simulink library "lka"  (Simulink 8.2)
settings: Solver=ode1  StartTime=0.0  StopTime=Inf  FixedStep=0.001  RelTol=1e-3
PostLoadFcn:
  | , if any(exist('dsrtsu_mdlpostloadfcn', 'file') == [2, 3, 6]), try dsrtsu_mdlpostloadfcn('Execute', bdroot); catch fprintf('Error in PostLoadFcn (dsrtsu_mdlpostloadfcn) for model "%s":\n %s\n', bdroot, lasterr); end, end,
undefined symbols (not defined in the file or in its folder): ALFC_VehSpd_X_kph, ALKA_LatSpd_X_mps, ALKA_VehSpd_X_kph, ENUM_LKASTATE_ADASFAILURE, ENUM_LKASTATE_DISABLED, ENUM_LKASTATE_EPSRECOVERYPENDING, ENUM_LKASTATE_LEFTASSISTING, ENUM_LKASTATE_OFF, ENUM_LKASTATE_OPERATIONAL, ENUM_LKASTATE_RIGHTASSISTING, ENUM_LKASTATE_STANDBY, FALSE, KAPP_StrCenterOffset_deg, KAPP_VehicleWidth_m, KAPP_Wheel2SteerRatio_rat, KAPP_WheelBase_m, KLKA_BaseTqReqMax_Nm, KLKA_BaseTqReqMin_Nm, KLKA_IGainLowerLimit_rad, KLKA_IGainUpperLimit_rad, KLKA_LKATqReqMax_Nm, KLKA_LKATqReqMin_Nm, KLKA_TargetPointShift_m, MLFC_KusCoeff_rat, MLKA_ControlGain_rat, MLKA_KgainRatio_rat, MLKA_LookAheadDist_Y_m, TRUE
libraries: hcu_lib x8, simulink x2
settings Model: DSRTSU_INTERNAL_RTI_VER=450  DSRTSU_INTERNAL_RTI_TYPE=rti1401  RTICANMMDATA=struct('GeneralSetupData',struct('modelroot','C:\ADAS\trunk\ADAS_Softwares\HTDragon\software\sw_development\arch\app\lka','generalsettings',struct('filesettings',struct('destfolder',struct('Name','RTICANMM_FILES','Check',1),'buildfolder',struct('Name','.','Check',1),'AbsDestfolder',struct('Name','C:\ADAS\trunk\ADAS_Softwares\HTDragon\software\sw_development\arch\app\lka\RTICANMM_FILES'),'AbsBuildfolder',struct('Name','C:\ADAS\trunk\ADAS_Softwares\HTDragon\software\sw_development\arch\app\lka'))),'options',struct('addpaths',1,'rmpaths',1,'addtrcexclusion',logical(1),'cannavigator',struct('checkmonitoring',0),'show_usrtrc',0,'use_usrtrc',0),'advanced',struct('options',[1 1 1 1 1 1 1 1 1 1 1 1 1 1 1 1 1 1 1 1 1 1 1 1 1 1 1 1 1 1 1 1 1 1 1 1 1 1 1 1 1 1 1 1 1 1 1 1 1 1 1 1 1 1 1 1 1 1 1 1 1 1 1 1 1 1 1 1 1 1 1 1 1 1 1 1 1 1 1 1 1 1 1 1 1 1 1 1 1 1 1 1 1 1 1 1 1 1 1 1]),'MPSetup',{{}},'modelname','lka','block','lka'))  DSRTSU_INTERNAL_RTIFPGA=40  Creator=14014  LastModifiedBy=13192

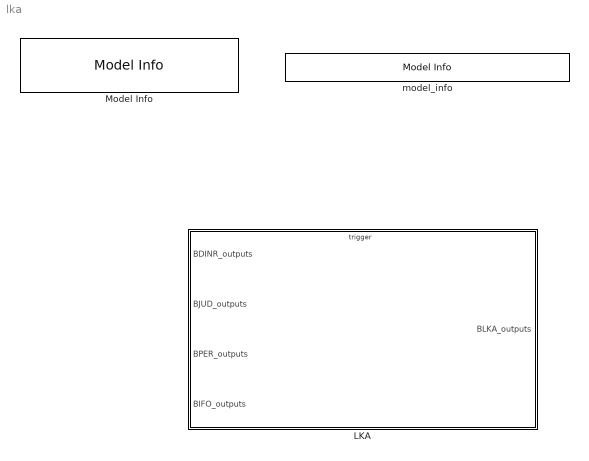
== system lka ==
  LKA : Subsystem
  Model Info : simulink/Model-Wide Utilities/Model Info  InitialBlockCM=None  BlockCM=None  Frame=on  DisplayStringWithTags=|  HorizontalTextAlignment=Left  LeftAlignmentValue=0.02  SourceBlockDiagram=lka  TagMaxNumber=20
      | Model Version        : %<ModelVersion>
      | Creator                   : %<Creator>
      | Last Modified by    : %<LastModifiedBy>
  model_info : simulink/Model-Wide Utilities/Model Info  InitialBlockCM=None  BlockCM=None  Frame=on  DisplayStringWithTags=$Id: lka.mdl 1622 2017-09-21 01:44:11Z bcluan $  HorizontalTextAlignment=Center  LeftAlignmentValue=0.5  SourceBlockDiagram=lka  TagMaxNumber=20

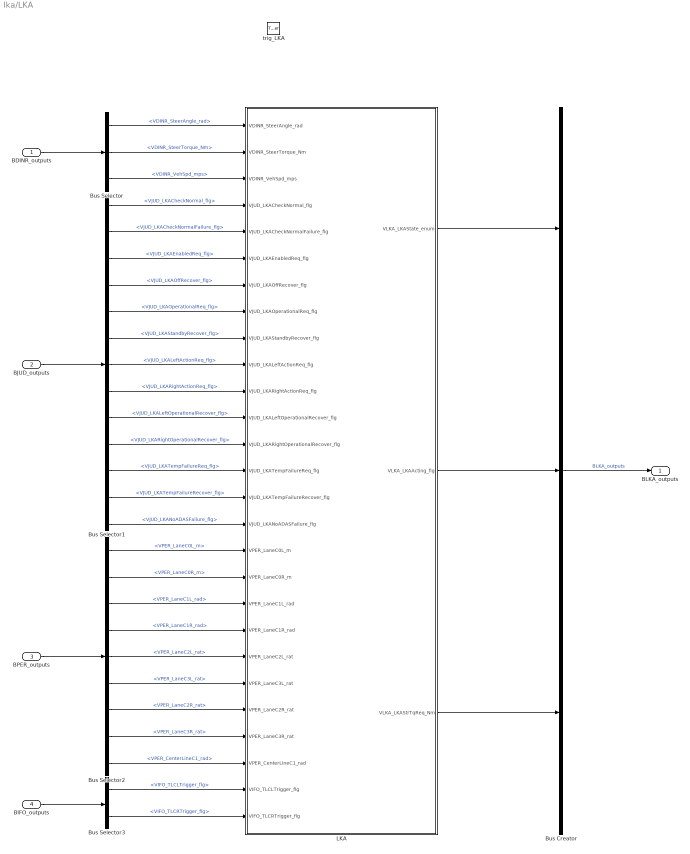
== system lka/LKA ==
  BDINR_outputs : Inport  OutDataTypeStr=Bus: BDINR_outputs
  BJUD_outputs : Inport  Port=2  OutDataTypeStr=Bus: BJUD_outputs
  BPER_outputs : Inport  Port=3  OutDataTypeStr=Bus: BPER_outputs
  BIFO_outputs : Inport  Port=4  OutDataTypeStr=Bus: BIFO_outputs
  trig_LKA : TriggerPort  TriggerType=function-call
      settings: AttributesFormatString=State = %<StatesWhenEnabling>
  Bus Creator : BusCreator  Inputs=3  OutDataTypeStr=Bus: BLKA_outputs
  Bus Selector : BusSelector  OutputSignals=VDINR_SteerAngle_rad,VDINR_SteerTorque_Nm,VDINR_VehSpd_mps
  Bus Selector1 : BusSelector  OutputSignals=VJUD_LKACheckNormal_flg,VJUD_LKACheckNormalFailure_flg,VJUD_LKAEnabledReq_flg,VJUD_LKAOffRecover_flg,VJUD_LKAOperationalReq_flg,VJUD_LKAStandbyRecover_flg,VJUD_LKALeftActionReq_flg,VJUD_LKARightActionReq_flg,VJUD_LKALeftOperationalRecover_flg,VJUD_LKARightOperationalRecover_flg,VJUD_LKATempFailureReq_flg,VJUD_LKATempFailureRecover_flg,VJUD_LKANoADASFailure_flg
  Bus Selector2 : BusSelector  OutputSignals=VPER_LaneC0L_m,VPER_LaneC0R_m,VPER_LaneC1L_rad,VPER_LaneC1R_rad,VPER_LaneC2L_rat,VPER_LaneC3L_rat,VPER_LaneC2R_rat,VPER_LaneC3R_rat,VPER_CenterLineC1_rad
  Bus Selector3 : BusSelector  OutputSignals=VIFO_TLCLTrigger_flg,VIFO_TLCRTrigger_flg
  LKA : Subsystem
  BLKA_outputs : Outport  OutDataTypeStr=Bus: BLKA_outputs
  wires:
  Bus Creator/1 -> BLKA_outputs/1  "BLKA_outputs"
  BDINR_outputs/1 -> Bus Selector/1
  BPER_outputs/1 -> Bus Selector2/1
  BJUD_outputs/1 -> Bus Selector1/1
  BIFO_outputs/1 -> Bus Selector3/1
  LKA/2(VLKA_LKAActing_flg) -> Bus Creator/2
  LKA/3(VLKA_LKAStrTqReq_Nm) -> Bus Creator/3
  LKA/1(VLKA_LKAState_enum) -> Bus Creator/1
  Bus Selector1/1 -> LKA/4(VJUD_LKACheckNormal_flg)  "<VJUD_LKACheckNormal_flg>"
  Bus Selector1/3 -> LKA/6(VJUD_LKAEnabledReq_flg)  "<VJUD_LKAEnabledReq_flg>"
  Bus Selector1/4 -> LKA/7(VJUD_LKAOffRecover_flg)  "<VJUD_LKAOffRecover_flg>"
  Bus Selector1/5 -> LKA/8(VJUD_LKAOperationalReq_flg)  "<VJUD_LKAOperationalReq_flg>"
  Bus Selector1/6 -> LKA/9(VJUD_LKAStandbyRecover_flg)  "<VJUD_LKAStandbyRecover_flg>"
  Bus Selector1/7 -> LKA/10(VJUD_LKALeftActionReq_flg)  "<VJUD_LKALeftActionReq_flg>"
  Bus Selector1/8 -> LKA/11(VJUD_LKARightActionReq_flg)  "<VJUD_LKARightActionReq_flg>"
  Bus Selector1/9 -> LKA/12(VJUD_LKALeftOperationalRecover_flg)  "<VJUD_LKALeftOperationalRecover_flg>"
  Bus Selector1/10 -> LKA/13(VJUD_LKARightOperationalRecover_flg)  "<VJUD_LKARightOperationalRecover_flg>"
  Bus Selector1/11 -> LKA/14(VJUD_LKATempFailureReq_flg)  "<VJUD_LKATempFailureReq_flg>"
  Bus Selector1/12 -> LKA/15(VJUD_LKATempFailureRecover_flg)  "<VJUD_LKATempFailureRecover_flg>"
  Bus Selector1/13 -> LKA/16(VJUD_LKANoADASFailure_flg)  "<VJUD_LKANoADASFailure_flg>"
  Bus Selector2/8 -> LKA/24(VPER_LaneC3R_rat)  "<VPER_LaneC3R_rat>"
  Bus Selector2/7 -> LKA/23(VPER_LaneC2R_rat)  "<VPER_LaneC2R_rat>"
  Bus Selector2/3 -> LKA/19(VPER_LaneC1L_rad)  "<VPER_LaneC1L_rad>"
  Bus Selector2/2 -> LKA/18(VPER_LaneC0R_m)  "<VPER_LaneC0R_m>"
  Bus Selector2/1 -> LKA/17(VPER_LaneC0L_m)  "<VPER_LaneC0L_m>"
  Bus Selector2/4 -> LKA/20(VPER_LaneC1R_rad)  "<VPER_LaneC1R_rad>"
  Bus Selector2/6 -> LKA/22(VPER_LaneC3L_rat)  "<VPER_LaneC3L_rat>"
  Bus Selector2/5 -> LKA/21(VPER_LaneC2L_rat)  "<VPER_LaneC2L_rat>"
  Bus Selector2/9 -> LKA/25(VPER_CenterLineC1_rad)  "<VPER_CenterLineC1_rad>"
  Bus Selector3/1 -> LKA/26(VIFO_TLCLTrigger_flg)  "<VIFO_TLCLTrigger_flg>"
  Bus Selector3/2 -> LKA/27(VIFO_TLCRTrigger_flg)  "<VIFO_TLCRTrigger_flg>"
  Bus Selector/1 -> LKA/1(VDINR_SteerAngle_rad)  "<VDINR_SteerAngle_rad>"
  Bus Selector/2 -> LKA/2(VDINR_SteerTorque_Nm)  "<VDINR_SteerTorque_Nm>"
  Bus Selector/3 -> LKA/3(VDINR_VehSpd_mps)  "<VDINR_VehSpd_mps>"
  Bus Selector1/2 -> LKA/5(VJUD_LKACheckNormalFailure_flg)  "<VJUD_LKACheckNormalFailure_flg>"

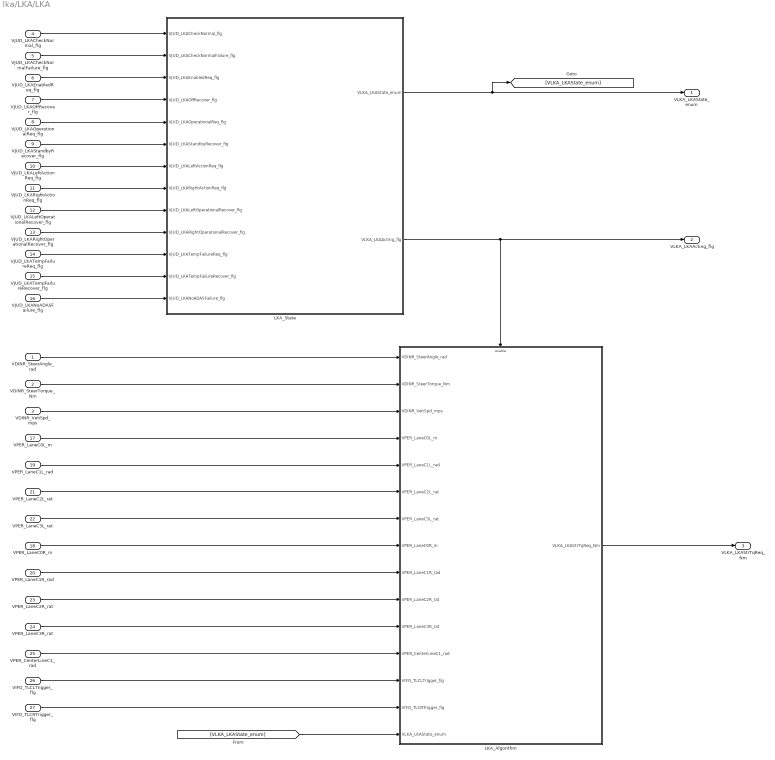
== system lka/LKA/LKA ==
  VDINR_SteerAngle_rad : Inport
  VDINR_SteerTorque_Nm : Inport  Port=2
  VDINR_VehSpd_mps : Inport  Port=3
  VJUD_LKACheckNormal_flg : Inport  Port=4
  VJUD_LKACheckNormalFailure_flg : Inport  Port=5
  VJUD_LKAEnabledReq_flg : Inport  Port=6
  VJUD_LKAOffRecover_flg : Inport  Port=7
  VJUD_LKAOperationalReq_flg : Inport  Port=8
  VJUD_LKAStandbyRecover_flg : Inport  Port=9
  VJUD_LKALeftActionReq_flg : Inport  Port=10
  VJUD_LKARightActionReq_flg : Inport  Port=11
  VJUD_LKALeftOperationalRecover_flg : Inport  Port=12
  VJUD_LKARightOperationalRecover_flg : Inport  Port=13
  VJUD_LKATempFailureReq_flg : Inport  Port=14
  VJUD_LKATempFailureRecover_flg : Inport  Port=15
  VJUD_LKANoADASFailure_flg : Inport  Port=16
  VPER_LaneC0L_m : Inport  Port=17
  VPER_LaneC0R_m : Inport  Port=18
  VPER_LaneC1L_rad : Inport  Port=19
  VPER_LaneC1R_rad : Inport  Port=20
  VPER_LaneC2L_rat : Inport  Port=21
  VPER_LaneC3L_rat : Inport  Port=22
  VPER_LaneC2R_rat : Inport  Port=23
  VPER_LaneC3R_rat : Inport  Port=24
  VPER_CenterLineC1_rad : Inport  Port=25
  VIFO_TLCLTrigger_flg : Inport  Port=26
  VIFO_TLCRTrigger_flg : Inport  Port=27
  LKA_Algorithm : Subsystem
  LKA_State : Stateflow chart  TreatAsAtomicUnit=on
  VLKA_LKAState_enum : Outport  OutputWhenDisabled=reset  InitialOutput=[0]
  VLKA_LKAActing_flg : Outport  Port=2  OutputWhenDisabled=reset  InitialOutput=[0]
  VLKA_LKAStrTqReq_Nm : Outport  Port=3  OutputWhenDisabled=reset  InitialOutput=[0]
  wires:
  VJUD_LKACheckNormal_flg/1 -> LKA_State/1(VJUD_LKACheckNormal_flg)
  VJUD_LKAEnabledReq_flg/1 -> LKA_State/3(VJUD_LKAEnabledReq_flg)
  VJUD_LKAOffRecover_flg/1 -> LKA_State/4(VJUD_LKAOffRecover_flg)
  VJUD_LKAOperationalReq_flg/1 -> LKA_State/5(VJUD_LKAOperationalReq_flg)
  VJUD_LKAStandbyRecover_flg/1 -> LKA_State/6(VJUD_LKAStandbyRecover_flg)
  VJUD_LKALeftActionReq_flg/1 -> LKA_State/7(VJUD_LKALeftActionReq_flg)
  VJUD_LKALeftOperationalRecover_flg/1 -> LKA_State/9(VJUD_LKALeftOperationalRecover_flg)
  VJUD_LKATempFailureReq_flg/1 -> LKA_State/11(VJUD_LKATempFailureReq_flg)
  VJUD_LKATempFailureRecover_flg/1 -> LKA_State/12(VJUD_LKATempFailureRecover_flg)
  VJUD_LKANoADASFailure_flg/1 -> LKA_State/13(VJUD_LKANoADASFailure_flg)
  LKA_State/1(VLKA_LKAState_enum) -> [VLKA_LKAState_enum], VLKA_LKAState_enum/1
  LKA_State/2(VLKA_LKAActing_flg) -> VLKA_LKAActing_flg/1, LKA_Algorithm/Enable
  LKA_Algorithm/1(VLKA_LKAStrTqReq_Nm) -> VLKA_LKAStrTqReq_Nm/1
  VDINR_VehSpd_mps/1 -> LKA_Algorithm/3(VDINR_VehSpd_mps)
  VIFO_TLCLTrigger_flg/1 -> LKA_Algorithm/13(VIFO_TLCLTrigger_fig)
  VIFO_TLCRTrigger_flg/1 -> LKA_Algorithm/14(VIFO_TLCRTrigger_fig)
  VDINR_SteerAngle_rad/1 -> LKA_Algorithm/1(VDINR_SteerAngle_rad)
  VDINR_SteerTorque_Nm/1 -> LKA_Algorithm/2(VDINR_SteerTorque_Nm)
  VJUD_LKARightActionReq_flg/1 -> LKA_State/8(VJUD_LKARightActionReq_flg)
  VJUD_LKARightOperationalRecover_flg/1 -> LKA_State/10(VJUD_LKARightOperationalRecover_flg)
  VPER_LaneC0L_m/1 -> LKA_Algorithm/4(VPER_LaneC0L_m)
  VPER_LaneC1L_rad/1 -> LKA_Algorithm/5(VPER_LaneC1L_rad)
  VPER_LaneC0R_m/1 -> LKA_Algorithm/8(VPER_LaneC0R_m)
  VPER_LaneC1R_rad/1 -> LKA_Algorithm/9(VPER_LaneC1R_rad)
  VPER_LaneC2L_rat/1 -> LKA_Algorithm/6(VPER_LaneC2L_rat)
  VPER_LaneC3L_rat/1 -> LKA_Algorithm/7(VPER_LaneC3L_rat)
  VPER_LaneC2R_rat/1 -> LKA_Algorithm/10(VPER_LaneC2R_rat)
  VPER_LaneC3R_rat/1 -> LKA_Algorithm/11(VPER_LaneC3R_rat)
  VPER_CenterLineC1_rad/1 -> LKA_Algorithm/12(VPER_CenterLineC1_rad)
  [VLKA_LKAState_enum] -> LKA_Algorithm/15(VLKA_LKAState_enum)
  VJUD_LKACheckNormalFailure_flg/1 -> LKA_State/2(VJUD_LKACheckNormalFailure_flg)

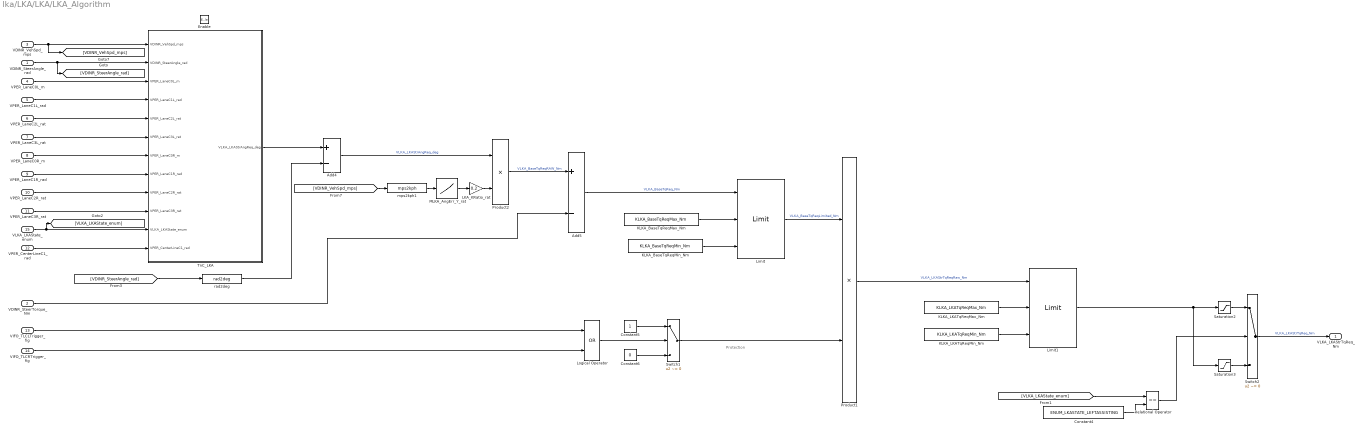
== system lka/LKA/LKA/LKA_Algorithm ==
  note: Protection
  VDINR_SteerAngle_rad : Inport
  VDINR_SteerTorque_Nm : Inport  Port=2
  VDINR_VehSpd_mps : Inport  Port=3
  VPER_LaneC0L_m : Inport  Port=4
  VPER_LaneC1L_rad : Inport  Port=5
  VPER_LaneC2L_rat : Inport  Port=6
  VPER_LaneC3L_rat : Inport  Port=7
  VPER_LaneC0R_m : Inport  Port=8
  VPER_LaneC1R_rad : Inport  Port=9
  VPER_LaneC2R_rat : Inport  Port=10
  VPER_LaneC3R_rat : Inport  Port=11
  VPER_CenterLineC1_rad : Inport  Port=12
  VIFO_TLCLTrigger_fig : Inport  Port=13
  VIFO_TLCRTrigger_fig : Inport  Port=14
  VLKA_LKAState_enum : Inport  Port=15
  Enable : EnablePort  StatesWhenEnabling=reset
  Add4 : Sum  Inputs=+-
  Add5 : Sum  Inputs=+-
  Constant4 : Constant  Value=ENUM_LKASTATE_LEFTASSISTING
  Constant5 : Constant  OutDataTypeStr=single
  Constant6 : Constant  Value=0  OutDataTypeStr=single
  KLKA_BaseTqReqMax_Nm : Constant  Value=KLKA_BaseTqReqMax_Nm  OutDataTypeStr=single
  KLKA_BaseTqReqMin_Nm : Constant  Value=KLKA_BaseTqReqMin_Nm  OutDataTypeStr=single
  KLKA_LKATqReqMax_Nm : Constant  Value=KLKA_LKATqReqMax_Nm  OutDataTypeStr=single
  KLKA_LKATqReqMin_Nm : Constant  Value=KLKA_LKATqReqMin_Nm  OutDataTypeStr=single
  LKA_KRatio_rat : Gain  Gain=0.2
  Limit : hcu_lib/Limit  SystemSampleTime=-1
  Limit1 : hcu_lib/Limit  SystemSampleTime=-1
  Logical Operator : Logic  Operator=OR  AllPortsSameDT=off  OutDataTypeStr=boolean
  MLKA_AngErr_Y_rat : Lookup  InputValues=[10:10:120]  Table=[1 1 1 1 1 1 1 1 1 1 1 1]  LookUpMeth=Interpolation-Use End Values
      settings: AttributesFormatString=%<InputValues>\n%<Table>
  Product1 : Product  RndMeth=Zero
  Product2 : Product
  Relational Operator : RelationalOperator  Operator===  OutDataTypeStr=boolean
  Saturation2 : Saturate  UpperLimit=0  LowerLimit=-inf
      settings: AttributesFormatString=|
      | %<UpperLimit>
      | %<LowerLimit>
  Saturation3 : Saturate  UpperLimit=inf  LowerLimit=0
      settings: AttributesFormatString=|
      | %<UpperLimit>
      | %<LowerLimit>
  Switch1 : Switch  Criteria=u2 ~= 0
  Switch2 : Switch  Criteria=u2 ~= 0
  TnC_LKA : Subsystem  TreatAsAtomicUnit=on
  mps2kph1 : hcu_lib/mps2kph
  rad2deg : hcu_lib/rad2deg
  VLKA_LKAStrTqReq_Nm : Outport  OutputWhenDisabled=reset  InitialOutput=[0]
  wires:
  Constant6/1 -> Switch1/3
  VIFO_TLCLTrigger_fig/1 -> Logical Operator/1
  VIFO_TLCRTrigger_fig/1 -> Logical Operator/2
  Logical Operator/1 -> Switch1/2
  Constant5/1 -> Switch1/1
  VDINR_SteerTorque_Nm/1 -> Add5/2
  VDINR_VehSpd_mps/1 -> [VDINR_VehSpd_mps], TnC_LKA/1(VDINR_VehSpd_mps)
  [VDINR_SteerAngle_rad] -> rad2deg/1
  TnC_LKA/1(VLKA_LKAStrAngReq_deg) -> Add4/1
  rad2deg/1 -> Add4/2
  Add4/1 -> Product2/1  "VLKA_LKAStrAngReq_deg"
  Product2/1 -> Add5/1  "VLKA_BaseTqReqRAW_Nm"
  Limit/1 -> Product1/1  "VLKA_BaseTqReqLimited_Nm"
  KLKA_BaseTqReqMax_Nm/1 -> Limit/2
  KLKA_BaseTqReqMin_Nm/1 -> Limit/3
  Add5/1 -> Limit/1  "VLKA_BaseTqReq_Nm"
  VDINR_SteerAngle_rad/1 -> [VDINR_SteerAngle_rad], TnC_LKA/2(VDINR_SteerAngle_rad)
  VPER_LaneC0L_m/1 -> TnC_LKA/3(VPER_LaneC0L_m)
  VPER_LaneC1L_rad/1 -> TnC_LKA/4(VPER_LaneC1L_rad)
  VPER_LaneC2L_rat/1 -> TnC_LKA/5(VPER_LaneC2L_rat)
  VPER_LaneC3L_rat/1 -> TnC_LKA/6(VPER_LaneC3L_rat)
  VPER_LaneC0R_m/1 -> TnC_LKA/7(VPER_LaneC0R_m)
  VPER_LaneC1R_rad/1 -> TnC_LKA/8(VPER_LaneC1R_rad)
  VPER_LaneC2R_rat/1 -> TnC_LKA/9(VPER_LaneC2R_rat)
  VPER_LaneC3R_rat/1 -> TnC_LKA/10(VPER_LaneC3R_rat)
  VLKA_LKAState_enum/1 -> [VLKA_LKAState_enum], TnC_LKA/11(VLKA_LKAState_enum)
  KLKA_LKATqReqMax_Nm/1 -> Limit1/2
  KLKA_LKATqReqMin_Nm/1 -> Limit1/3
  Product1/1 -> Limit1/1  "VLKA_LKAStrTqReqRaw_Nm"
  MLKA_AngErr_Y_rat/1 -> LKA_KRatio_rat/1
  mps2kph1/1 -> MLKA_AngErr_Y_rat/1
  [VDINR_VehSpd_mps] -> mps2kph1/1
  VPER_CenterLineC1_rad/1 -> TnC_LKA/12(VPER_CenterLineC1_rad)
  Switch1/1 -> Product1/2
  LKA_KRatio_rat/1 -> Product2/2
  Limit1/1 -> Saturation3/1, Saturation2/1
  Saturation2/1 -> Switch2/1
  Saturation3/1 -> Switch2/3
  Switch2/1 -> VLKA_LKAStrTqReq_Nm/1  "VLKA_LKAStrTqReq_Nm"
  [VLKA_LKAState_enum] -> Relational Operator/1
  Constant4/1 -> Relational Operator/2
  Relational Operator/1 -> Switch2/2

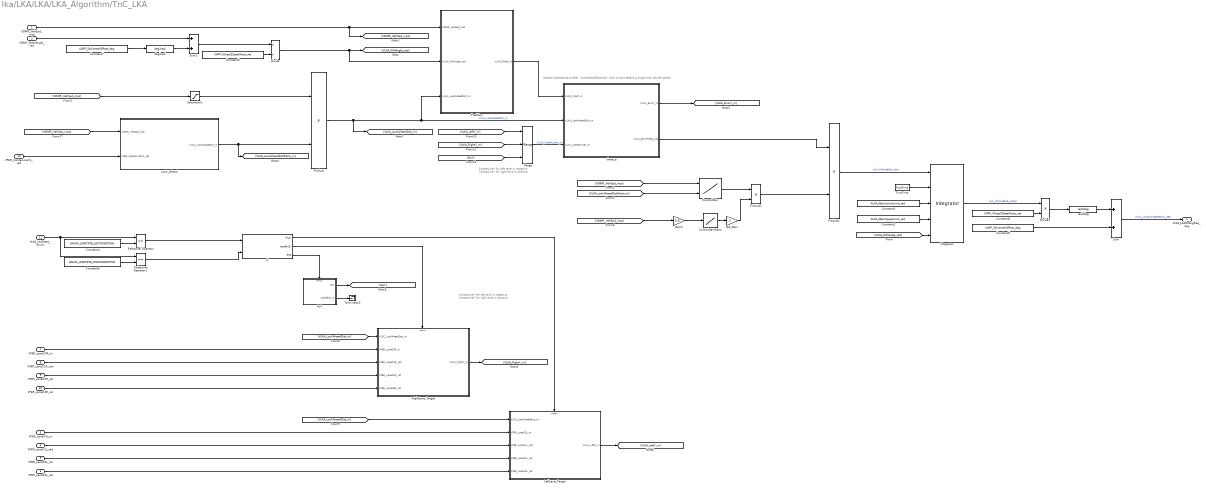
== system lka/LKA/LKA/LKA_Algorithm/TnC_LKA ==
  note: CenterLineY for left lane is negative
      | CenterLineY for right lane is positive
  note: Lateral displacement after "LookAheadDistance" with current steering angle and vehicle speed
  note: CenterLineY for left lane is negative
      | CenterLineY for right lane is positive
  VDINR_VehSpd_mps : Inport
  VDINR_SteerAngle_rad : Inport  Port=2
  VPER_LaneC0L_m : Inport  Port=3
  VPER_LaneC1L_rad : Inport  Port=4
  VPER_LaneC2L_rat : Inport  Port=5
  VPER_LaneC3L_rat : Inport  Port=6
  VPER_LaneC0R_m : Inport  Port=7
  VPER_LaneC1R_rad : Inport  Port=8
  VPER_LaneC2R_rat : Inport  Port=9
  VPER_LaneC3R_rat : Inport  Port=10
  VLKA_LKAState_enum : Inport  Port=11
  VPER_CenterLineC1_rad : Inport  Port=12
  Constant1 : Constant  Value=KLKA_IGainLowerLimit_rad
  Constant2 : Constant  Value=KLKA_IGainUpperLimit_rad
  Constant3 : Constant  Value=KAPP_Wheel2SteerRatio_rat
  Constant4 : Constant  Value=ENUM_LKASTATE_LEFTASSISTING
  Constant5 : Constant  Value=KAPP_StrCenterOffset_deg
  Constant6 : Constant  Value=ENUM_LKASTATE_RIGHTASSISTING
  Constant7 : Constant  Value=KAPP_StrCenterOffset_deg
  Constant8 : Constant  Value=KAPP_Wheel2SteerRatio_rat
  ControlGain : Lookup2D  RowIndex=ALKA_VehSpd_X_mps  ColumnIndex=ALKA_LookAheadDist_Y_m  Table=MLKA_ControlGain_rat  LookUpMeth=Interpolation-Use End Values  OutDataTypeStr=single
      settings: AttributesFormatString=|
      | <row=%<RowIndex>>
      | <column=%<ColumnIndex>>
      | <table=%<Table>>
  ControlGainRatio : Lookup  InputValues=ALKA_VehSpd_X_kph  Table=MLKA_KgainRatio_rat  LookUpMeth=Interpolation-Use End Values
      settings: AttributesFormatString=%<InputValues>\n%<Table>
  Divide : Product  Inputs=*/
  Divide1 : Product  Inputs=**
  FirstTime : hcu_lib/FirstTime
  Gain3 : Gain  Gain=3.6
  If : If  NumInputs=2  IfExpression=u1  ElseIfExpressions=u2
  Integrator : hcu_lib/Integrator  SystemSampleTime=-1
  LKA_Gain : Gain
  LeftLane_Target : Subsystem  TreatAsAtomicUnit=on
  Look_Ahead : Subsystem
  Merge : Merge  Inputs=3
  NoY : Subsystem  TreatAsAtomicUnit=on
  Predition : Subsystem  TreatAsAtomicUnit=on
  Product : Product  RndMeth=Zero
  Product1 : Product  RndMeth=Zero
  Product2 : Product  RndMeth=Zero
  Relational Operator : RelationalOperator  Operator===  OutDataTypeStr=boolean
  Relational Operator1 : RelationalOperator  Operator===  OutDataTypeStr=boolean
  RightLane_Target : Subsystem  TreatAsAtomicUnit=on
  Saturation1 : Saturate  UpperLimit=41.66  LowerLimit=2.78
      settings: AttributesFormatString=upper = %<UpperLimit>\nlower = %<LowerLimit>
  Sum : Sum
  Sum1 : Sum
  Terminator1 : Terminator
  deg2rad : hcu_lib/deg2rad
  rad2deg : hcu_lib/rad2deg
  theta_e : Subsystem  TreatAsAtomicUnit=on
  VLKA_LKAStrAngReq_deg : Outport  OutputWhenDisabled=reset  InitialOutput=[0]
  wires:
  Constant2/1 -> Integrator/4
  Constant1/1 -> Integrator/3
  rad2deg/1 -> Sum/1
  Predition/1(VLKA_PredY_m) -> theta_e/1(VLKA_PredY_m)
  [VLKA_WhlAngle_rad] -> Integrator/5
  VDINR_SteerAngle_rad/1 -> Sum1/1
  Divide1/1 -> rad2deg/1
  theta_e/1(VLKA_ErrorY_m) -> [VLKA_ErrorY_m]
  VDINR_VehSpd_mps/1 -> [VDINR_VehSpd_mps], Predition/1(VDINR_VehSpd_mps)
  Product1/1 -> Integrator/1  "LKA_WhlAngRad_input"
  Divide/1 -> Predition/2(VLKA_WhlAngle_rad), [VLKA_WhlAngle_rad]
  FirstTime/1 -> Integrator/2
  Constant5/1 -> Sum/2
  Sum/1 -> VLKA_LKAStrAngReq_deg/1  "VLKA_LKAStrAngReqRAW_deg"
  Integrator/1 -> Divide1/1  "LKA_WhlAngRad_output"
  Constant7/1 -> deg2rad/1
  deg2rad/1 -> Sum1/2
  Sum1/1 -> Divide/1
  [VDINR_VehSpd_mps] -> Saturation1/1
  [VDINR_VehSpd_mps] -> ControlGain/1
  [VLKA_LookAheadDistRatio_m] -> ControlGain/2
  [VDINR_VehSpd_mps] -> Gain3/1
  Gain3/1 -> ControlGainRatio/1
  Saturation1/1 -> Product/1
  Product/1 -> [VLKA_LookAheadDist_m], Predition/3(VLKA_LookAheadDist_m), theta_e/2(VLKA_LookAheadDist_m)  "VLKA_LookAheadDist_m"
  ControlGain/1 -> Product2/1
  ControlGainRatio/1 -> LKA_Gain/1
  VLKA_LKAState_enum/1 -> Relational Operator1/1, Relational Operator/1
  Constant4/1 -> Relational Operator/2
  Relational Operator/1 -> If/1
  Constant6/1 -> Relational Operator1/2
  Relational Operator1/1 -> If/2
  If/1 -> LeftLane_Target/Action
  If/2 -> RightLane_Target/Action
  [VLKA_LookAheadDist_m] -> RightLane_Target/1(VLFC_LookAheadDist_m)
  [VLKA_LookAheadDist_m] -> LeftLane_Target/1(VLFC_LookAheadDist_m)
  VPER_LaneC0L_m/1 -> LeftLane_Target/2(VPER_LaneC0L_m)
  VPER_LaneC1L_rad/1 -> LeftLane_Target/3(VPER_LaneC1L_rad)
  VPER_LaneC2L_rat/1 -> LeftLane_Target/4(VPER_LaneC2L_rat)
  VPER_LaneC3L_rat/1 -> LeftLane_Target/5(VPER_LaneC3L_rat)
  VPER_LaneC1R_rad/1 -> RightLane_Target/3(VPER_LaneC1R_rad)
  VPER_LaneC0R_m/1 -> RightLane_Target/2(VPER_LaneC0R_m)
  VPER_LaneC2R_rat/1 -> RightLane_Target/4(VPER_LaneC2R_rat)
  VPER_LaneC3R_rat/1 -> RightLane_Target/5(VPER_LaneC3R_rat)
  If/3 -> NoY/Action
  RightLane_Target/1(VLKA_RightY_m) -> [VLKA_RightY_m]
  LeftLane_Target/1(VLKA_LeftY_m) -> [VLKA_LeftY_m]
  Merge/1 -> theta_e/3(VLKA_CenterLineY_m)  "VLKA_CneterLIineY_m"
  [VLKA_LeftY_m] -> Merge/1
  [VLKA_RightY_m] -> Merge/2
  [NoY] -> Merge/3
  NoY/1(NoY) -> [NoY]
  NoY/2(C0Offset_m) -> Terminator1/1
  Constant3/1 -> Divide/2
  Product2/1 -> Product1/2
  Constant8/1 -> Divide1/2
  [VDINR_VehSpd_mps] -> Look_Ahead/1(VDINR_VehSpd_mps)
  VPER_CenterLineC1_rad/1 -> Look_Ahead/2(VPER_CenterLineC1_rad)
  theta_e/2(VLKA_ErrorTheta_rad) -> Product1/1
  Look_Ahead/1(VLKA_LookAheadDist_m) -> [VLKA_LookAheadDistRatio_m], Product/2
  LKA_Gain/1 -> Product2/2

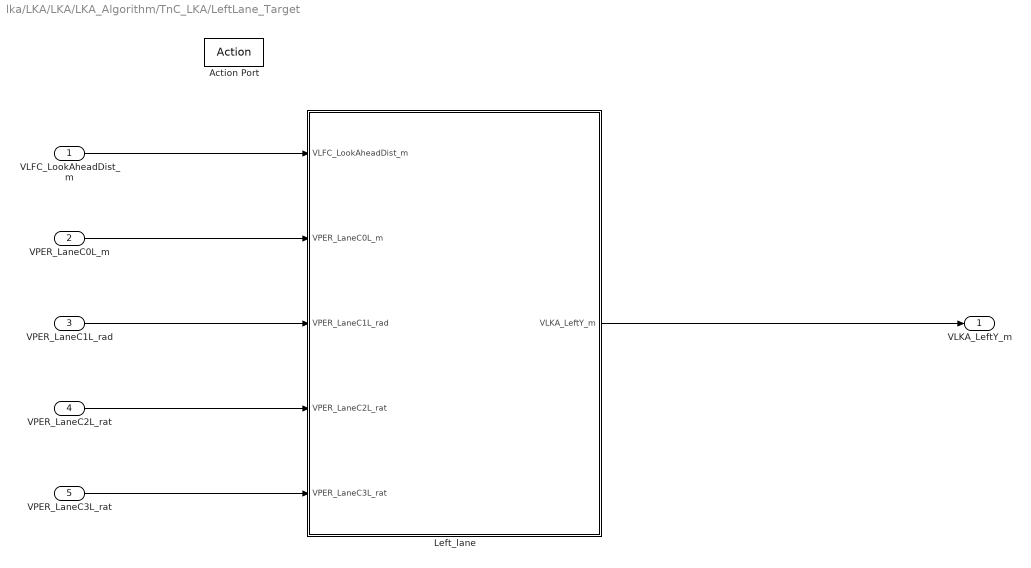
== system lka/LKA/LKA/LKA_Algorithm/TnC_LKA/LeftLane_Target ==
  VLFC_LookAheadDist_m : Inport
  VPER_LaneC0L_m : Inport  Port=2
  VPER_LaneC1L_rad : Inport  Port=3
  VPER_LaneC2L_rat : Inport  Port=4
  VPER_LaneC3L_rat : Inport  Port=5
  Action Port : ActionPort  InitializeStates=reset  ActionType=then
  Left_lane : Subsystem  TreatAsAtomicUnit=on
  VLKA_LeftY_m : Outport  OutputWhenDisabled=reset  InitialOutput=[0]
  wires:
  VPER_LaneC1L_rad/1 -> Left_lane/3(VPER_LaneC1L_rad)
  VPER_LaneC2L_rat/1 -> Left_lane/4(VPER_LaneC2L_rat)
  VPER_LaneC3L_rat/1 -> Left_lane/5(VPER_LaneC3L_rat)
  VLFC_LookAheadDist_m/1 -> Left_lane/1(VLFC_LookAheadDist_m)
  Left_lane/1(VLKA_LeftY_m) -> VLKA_LeftY_m/1
  VPER_LaneC0L_m/1 -> Left_lane/2(VPER_LaneC0L_m)

== system lka/LKA/LKA/LKA_Algorithm/TnC_LKA/Look_Ahead ==
  VDINR_VehSpd_mps : Inport
  VPER_CenterLineC1_rad : Inport  Port=2
  Abs2 : Abs
  MLKA_LatSpdTqComp_Y_rat : Lookup  InputValues=ALKA_LatSpd_X_mps  Table=MLKA_LookAheadDist_Y_m  LookUpMeth=Interpolation-Use End Values
      settings: AttributesFormatString=%<InputValues>\n%<Table>
  Product3 : Product
  VLKA_LookAheadDist_m : Outport
  wires:
  VDINR_VehSpd_mps/1 -> Product3/1
  VPER_CenterLineC1_rad/1 -> Product3/2
  Product3/1 -> Abs2/1
  Abs2/1 -> MLKA_LatSpdTqComp_Y_rat/1  "VLKA_LatSpd_kph"
  MLKA_LatSpdTqComp_Y_rat/1 -> VLKA_LookAheadDist_m/1

== system lka/LKA/LKA/LKA_Algorithm/TnC_LKA/NoY ==
  Action Port : ActionPort  InitializeStates=reset  ActionType=else
  Constant : Constant  Value=single(0)
  Constant1 : Constant  Value=single(0)
  NoY : Outport  OutputWhenDisabled=reset  InitialOutput=[0]
  C0Offset_m : Outport  Port=2  OutputWhenDisabled=reset  InitialOutput=[0]
  wires:
  Constant/1 -> NoY/1
  Constant1/1 -> C0Offset_m/1

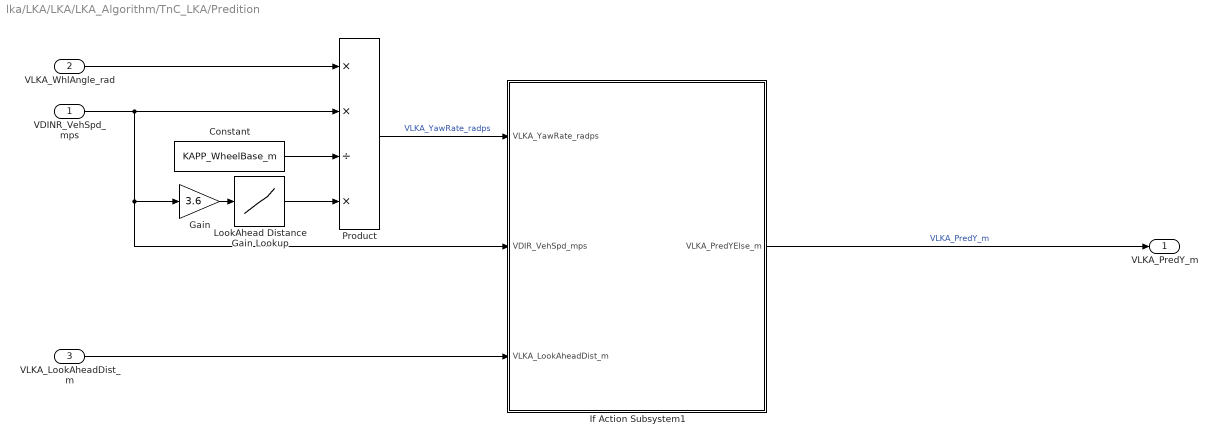
== system lka/LKA/LKA/LKA_Algorithm/TnC_LKA/Predition ==
  VDINR_VehSpd_mps : Inport
  VLKA_WhlAngle_rad : Inport  Port=2
  VLKA_LookAheadDist_m : Inport  Port=3
  Constant : Constant  Value=KAPP_WheelBase_m
  Gain : Gain  Gain=3.6  ParamDataTypeStr=single
  If Action Subsystem1 : Subsystem  TreatAsAtomicUnit=on
  LookAhead Distance Gain Lookup : Lookup  InputValues=ALFC_VehSpd_X_kph  Table=MLFC_KusCoeff_rat  LookUpMeth=Interpolation-Use End Values
      settings: AttributesFormatString=%<InputValues>\n%<Table>
  Product : Product  Inputs=**/*  RndMeth=Zero
  VLKA_PredY_m : Outport
  wires:
  Gain/1 -> LookAhead Distance Gain Lookup/1
  LookAhead Distance Gain Lookup/1 -> Product/4
  Product/1 -> If Action Subsystem1/1(VLKA_YawRate_radps)  "VLKA_YawRate_radps"
  VLKA_WhlAngle_rad/1 -> Product/1
  VDINR_VehSpd_mps/1 -> Gain/1, If Action Subsystem1/2(VDIR_VehSpd_mps), Product/2
  Constant/1 -> Product/3
  VLKA_LookAheadDist_m/1 -> If Action Subsystem1/3(VLKA_LookAheadDist_m)
  If Action Subsystem1/1(VLKA_PredYElse_m) -> VLKA_PredY_m/1  "VLKA_PredY_m"

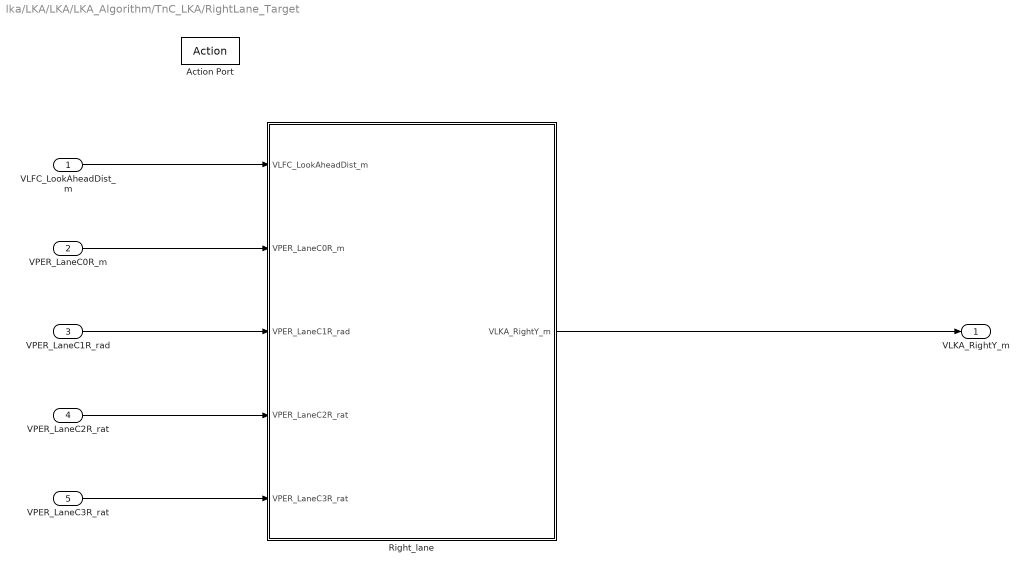
== system lka/LKA/LKA/LKA_Algorithm/TnC_LKA/RightLane_Target ==
  VLFC_LookAheadDist_m : Inport
  VPER_LaneC0R_m : Inport  Port=2
  VPER_LaneC1R_rad : Inport  Port=3
  VPER_LaneC2R_rat : Inport  Port=4
  VPER_LaneC3R_rat : Inport  Port=5
  Action Port : ActionPort  InitializeStates=reset  ActionType=elseif
  Right_lane : Subsystem  TreatAsAtomicUnit=on
  VLKA_RightY_m : Outport  OutputWhenDisabled=reset  InitialOutput=[0]
  wires:
  VPER_LaneC1R_rad/1 -> Right_lane/3(VPER_LaneC1R_rad)
  VPER_LaneC2R_rat/1 -> Right_lane/4(VPER_LaneC2R_rat)
  VPER_LaneC3R_rat/1 -> Right_lane/5(VPER_LaneC3R_rat)
  Right_lane/1(VLKA_RightY_m) -> VLKA_RightY_m/1
  VLFC_LookAheadDist_m/1 -> Right_lane/1(VLFC_LookAheadDist_m)
  VPER_LaneC0R_m/1 -> Right_lane/2(VPER_LaneC0R_m)

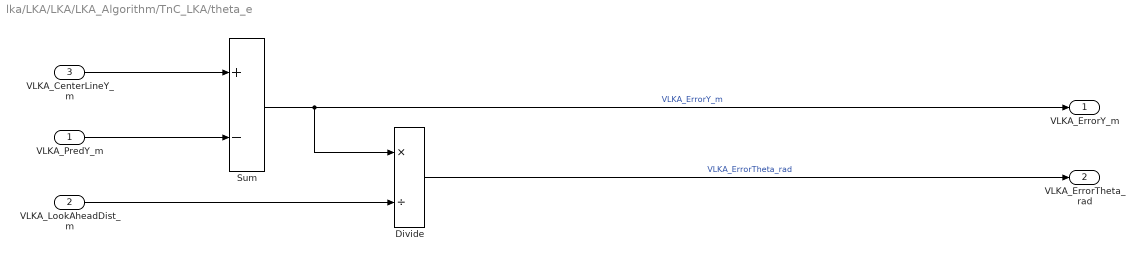
== system lka/LKA/LKA/LKA_Algorithm/TnC_LKA/theta_e ==
  VLKA_PredY_m : Inport
  VLKA_LookAheadDist_m : Inport  Port=2
  VLKA_CenterLineY_m : Inport  Port=3
  Divide : Product  Inputs=*/
  Sum : Sum  Inputs=+-
  VLKA_ErrorY_m : Outport
  VLKA_ErrorTheta_rad : Outport  Port=2
  wires:
  Divide/1 -> VLKA_ErrorTheta_rad/1  "VLKA_ErrorTheta_rad"
  VLKA_LookAheadDist_m/1 -> Divide/2
  Sum/1 -> Divide/1, VLKA_ErrorY_m/1  "VLKA_ErrorY_m"
  VLKA_CenterLineY_m/1 -> Sum/1
  VLKA_PredY_m/1 -> Sum/2

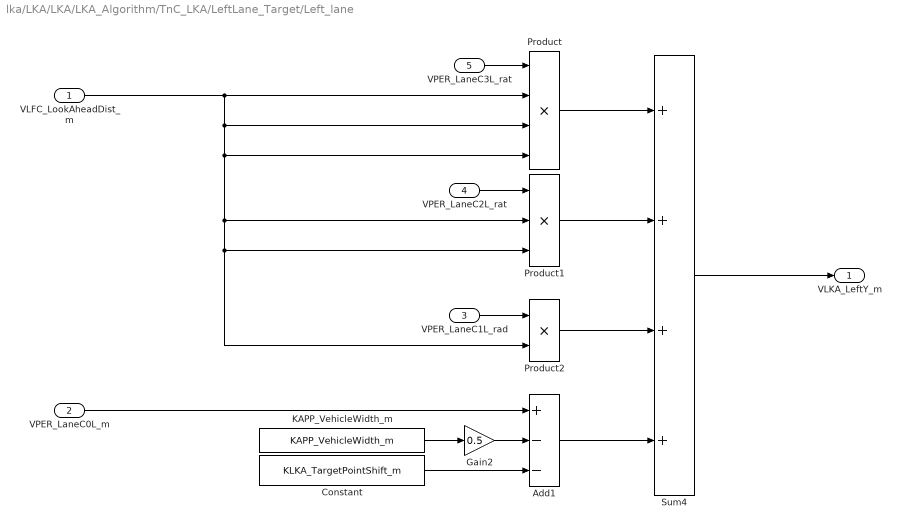
== system lka/LKA/LKA/LKA_Algorithm/TnC_LKA/LeftLane_Target/Left_lane ==
  VLFC_LookAheadDist_m : Inport
  VPER_LaneC0L_m : Inport  Port=2
  VPER_LaneC1L_rad : Inport  Port=3
  VPER_LaneC2L_rat : Inport  Port=4
  VPER_LaneC3L_rat : Inport  Port=5
  Add1 : Sum  Inputs=+--
  Constant : Constant  Value=KLKA_TargetPointShift_m
  Gain2 : Gain  Gain=0.5
  "KAPP_VehicleWidth_m " : Constant  Value=KAPP_VehicleWidth_m
  Product : Product  Inputs=4  RndMeth=Zero
  Product1 : Product  Inputs=3  RndMeth=Zero
  Product2 : Product  RndMeth=Zero
  Sum4 : Sum  Inputs=++++
  VLKA_LeftY_m : Outport
  wires:
  VPER_LaneC0L_m/1 -> Add1/1
  Product2/1 -> Sum4/3
  Product1/1 -> Sum4/2
  Product/1 -> Sum4/1
  VPER_LaneC1L_rad/1 -> Product2/1
  VPER_LaneC2L_rat/1 -> Product1/1
  VPER_LaneC3L_rat/1 -> Product/1
  VLFC_LookAheadDist_m/1 -> Product/2, Product/3, Product/4, Product1/2, Product2/2, Product1/3
  Sum4/1 -> VLKA_LeftY_m/1
  "KAPP_VehicleWidth_m "/1 -> Gain2/1
  Gain2/1 -> Add1/2
  Add1/1 -> Sum4/4
  Constant/1 -> Add1/3

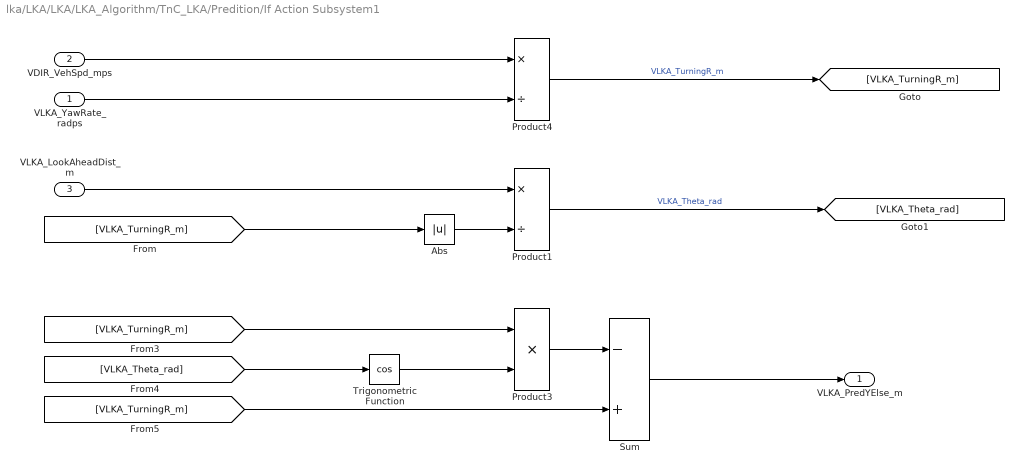
== system lka/LKA/LKA/LKA_Algorithm/TnC_LKA/Predition/If Action Subsystem1 ==
  VLKA_YawRate_radps : Inport
  VDIR_VehSpd_mps : Inport  Port=2
  VLKA_LookAheadDist_m : Inport  Port=3
  Abs : Abs
  Product1 : Product  Inputs=*/  RndMeth=Zero
  Product3 : Product  Inputs=**  RndMeth=Zero
  Product4 : Product  Inputs=*/  RndMeth=Zero
  Sum : Sum  Inputs=-+
  Trigonometric Function : Trigonometry  Operator=cos
  VLKA_PredYElse_m : Outport
  wires:
  Trigonometric Function/1 -> Product3/2
  Abs/1 -> Product1/2
  VDIR_VehSpd_mps/1 -> Product4/1
  VLKA_YawRate_radps/1 -> Product4/2
  VLKA_LookAheadDist_m/1 -> Product1/1
  Product4/1 -> [VLKA_TurningR_m]  "VLKA_TurningR_m"
  [VLKA_TurningR_m] -> Abs/1
  Product1/1 -> [VLKA_Theta_rad]  "VLKA_Theta_rad"
  [VLKA_TurningR_m] -> Product3/1
  [VLKA_Theta_rad] -> Trigonometric Function/1
  Product3/1 -> Sum/1
  [VLKA_TurningR_m] -> Sum/2
  Sum/1 -> VLKA_PredYElse_m/1

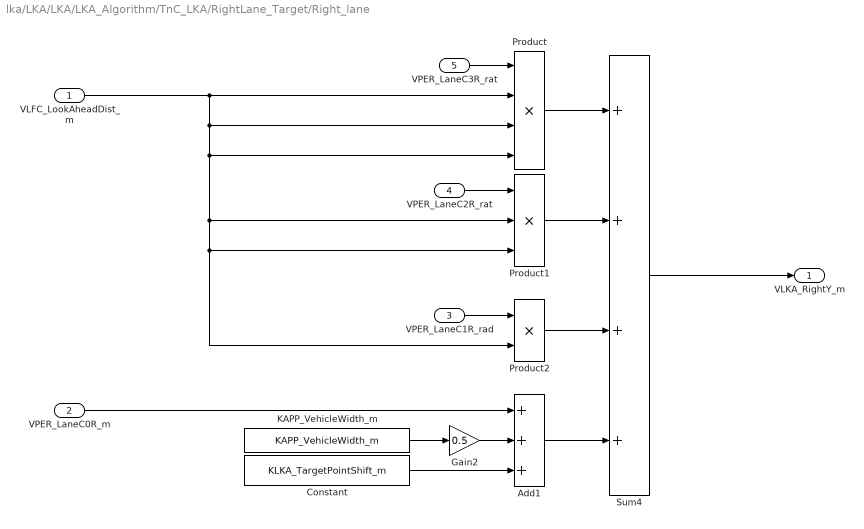
== system lka/LKA/LKA/LKA_Algorithm/TnC_LKA/RightLane_Target/Right_lane ==
  VLFC_LookAheadDist_m : Inport
  VPER_LaneC0R_m : Inport  Port=2
  VPER_LaneC1R_rad : Inport  Port=3
  VPER_LaneC2R_rat : Inport  Port=4
  VPER_LaneC3R_rat : Inport  Port=5
  Add1 : Sum  Inputs=+++
  Constant : Constant  Value=KLKA_TargetPointShift_m
  Gain2 : Gain  Gain=0.5
  "KAPP_VehicleWidth_m " : Constant  Value=KAPP_VehicleWidth_m
  Product : Product  Inputs=4  RndMeth=Zero
  Product1 : Product  Inputs=3  RndMeth=Zero
  Product2 : Product  RndMeth=Zero
  Sum4 : Sum  Inputs=++++
  VLKA_RightY_m : Outport
  wires:
  Product2/1 -> Sum4/3
  Product1/1 -> Sum4/2
  Product/1 -> Sum4/1
  VPER_LaneC1R_rad/1 -> Product2/1
  VPER_LaneC2R_rat/1 -> Product1/1
  VPER_LaneC3R_rat/1 -> Product/1
  VLFC_LookAheadDist_m/1 -> Product/2, Product/3, Product/4, Product1/2, Product2/2, Product1/3
  Sum4/1 -> VLKA_RightY_m/1
  "KAPP_VehicleWidth_m "/1 -> Gain2/1
  Gain2/1 -> Add1/2
  Constant/1 -> Add1/3
  VPER_LaneC0R_m/1 -> Add1/1
  Add1/1 -> Sum4/4

== stateflow chart LKA/LKA/LKA_State ==
  state NORMAL
    state DISABLED
      en:
      VLKA_LKAState_enum=ENUM_LKASTATE_DISABLED;
      VLKA_LKAActing_flg = FALSE;
    state ENABLED
      state ON
        state ACTIVE
          state OPERATIONAL
            en:
            VLKA_LKAState_enum=ENUM_LKASTATE_OPERATIONAL;
            VLKA_LKAActing_flg = FALSE;
          state LEFT_ASSIST
            en:
            VLKA_LKAState_enum=ENUM_LKASTATE_LEFTASSISTING;
            VLKA_LKAActing_flg = TRUE;
          state RIGHT_ASSIST
            en:
            VLKA_LKAState_enum=ENUM_LKASTATE_RIGHTASSISTING;
            VLKA_LKAActing_flg = TRUE;
          (default) -> OPERATIONAL
          OPERATIONAL -> LEFT_ASSIST [order 1] : [VJUD_LKALeftActionReq_flg]
          LEFT_ASSIST -> OPERATIONAL : [VJUD_LKALeftOperationalRecover_flg]
          OPERATIONAL -> RIGHT_ASSIST [order 2] : [VJUD_LKARightActionReq_flg]
          RIGHT_ASSIST -> OPERATIONAL : [VJUD_LKARightOperationalRecover_flg]
        state STANDBY
          en:
          VLKA_LKAState_enum=ENUM_LKASTATE_STANDBY;
          VLKA_LKAActing_flg = FALSE;
        (default) -> STANDBY
        STANDBY -> ACTIVE : [VJUD_LKAOperationalReq_flg]
        ACTIVE -> STANDBY : [VJUD_LKAStandbyRecover_flg]
      state OFF
        en:
        VLKA_LKAState_enum=ENUM_LKASTATE_OFF;
        VLKA_LKAActing_flg = FALSE;
      (default) -> OFF
      OFF -> ON : [VJUD_LKAEnabledReq_flg]
      ON -> OFF : [VJUD_LKAOffRecover_flg]
    (default) -> DISABLED
    DISABLED -> ENABLED : [VJUD_LKACheckNormal_flg]
    ENABLED -> DISABLED : [VJUD_LKACheckNormalFailure_flg]
  state FAILURE_TEMPORARY
    state ADAS_FAILURE
      en:
      VLKA_LKAState_enum=ENUM_LKASTATE_ADASFAILURE;
      VLKA_LKAActing_flg = FALSE;
    state EPS_FAILURE
      en:
      VLKA_LKAState_enum=ENUM_LKASTATE_EPSRECOVERYPENDING;
      VLKA_LKAActing_flg = FALSE;
    (default) -> ADAS_FAILURE
    ADAS_FAILURE -> EPS_FAILURE : [VJUD_LKANoADASFailure_flg]
    EPS_FAILURE -> ADAS_FAILURE : [!VJUD_LKANoADASFailure_flg]
  (default) -> NORMAL
  NORMAL -> FAILURE_TEMPORARY : [VJUD_LKATempFailureReq_flg]
  FAILURE_TEMPORARY -> NORMAL : [VJUD_LKATempFailureRecover_flg]
  data: TRUE parameter double; FALSE parameter double; ENUM_LKASTATE_DISABLED parameter double; ENUM_LKASTATE_OFF parameter double; ENUM_LKASTATE_STANDBY parameter double; ENUM_LKASTATE_OPERATIONAL parameter double; ENUM_LKASTATE_RIGHTASSISTING parameter double; ENUM_LKASTATE_ADASFAILURE parameter double; ENUM_LKASTATE_EPSRECOVERYPENDING parameter double; VLKA_LKAState_enum output double; VLKA_LKAActing_flg output double; VJUD_LKACheckNormal_flg input double; VJUD_LKACheckNormalFailure_flg input double; VJUD_LKAEnabledReq_flg input double; VJUD_LKAOffRecover_flg input double; VJUD_LKAOperationalReq_flg input double; VJUD_LKAStandbyRecover_flg input double; VJUD_LKALeftActionReq_flg input double; VJUD_LKARightActionReq_flg input double; VJUD_LKALeftOperationalRecover_flg input double; VJUD_LKARightOperationalRecover_flg input double; VJUD_LKATempFailureReq_flg input double; VJUD_LKATempFailureRecover_flg input double; VJUD_LKANoADASFailure_flg input double; ENUM_LKASTATE_LEFTASSISTING parameter double
